simulink model "test1"  (Simulink 10.0)
settings: Solver=VariableStepAuto  StartTime=0.0  StopTime=10.0  RelTol=1e-3
settings Model: Creator=Tan Eng Meng  LastModifiedBy=Tan Eng Meng
settings DataIOCC: SaveFormat=Dataset  ReturnWorkspaceOutputs=on
settings OptimizationCC: LifeSpan=auto
settings DebuggingCC: UnderspecifiedInitializationDetection=Simplified  MergeDetectMultiDrivingBlocksExec=error  SFUnexpectedBacktrackingDiag=error  SFNoUnconditionalDefaultTransitionDiag=error  SFExecutionAtInitializationDiag=warning  ArithmeticOperatorsInVariantConditions=error
settings HardwareCC: ProdBitPerPointer=64  ProdBitPerSizeT=64  ProdBitPerPtrDiffT=64  ProdLargestAtomicFloat=Float  ProdIntDivRoundTo=Zero  ProdEndianess=LittleEndian  ProdWordSize=64  ProdHWDeviceType=Intel->x86-64 (Windows64)
settings ModelReferenceCC: PropagateSignalLabelsOutOfModel=on
settings SFSimCC: SimUseLocalCustomCode=on  CustomCodeUndefinedFunction=FilterOut
settings RTWCC: RTWUseLocalCustomCode=on
settings CodeAppCC: StateflowObjectComments=off
settings GRTTargetCC: TargetLangStandard=C99 (ISO)  CombineOutputUpdateFcns=on  GRTInterface=off
settings ConfigComp: CovMetricSettings=dwe  CovHtmlReporting=off  CovSaveCumulativeToWorkspaceVar=off  CovSaveSingleToWorkspaceVar=off

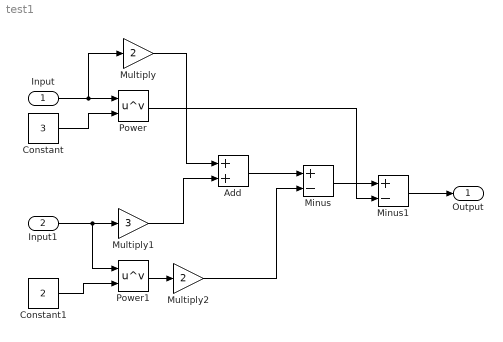
== system test1 ==
  Input : Inport
  Input1 : Inport  Port=2
  Add : Sum
  Constant : Constant  Value=3
  Constant1 : Constant  Value=2
  Minus : Sum  Inputs=+-
  Minus1 : Sum  Inputs=+-
  Multiply : Gain  Gain=2
  Multiply1 : Gain  Gain=3
  Multiply2 : Gain  Gain=2
  Power : Math  Operator=pow  SignedPower=off  SaturateOnIntegerOverflow=on
  Power1 : Math  Operator=pow  SignedPower=off  SaturateOnIntegerOverflow=on
  Output : Outport
  wires:
  Input/1 -> Multiply/1, Power/1
  Constant/1 -> Power/2
  Input1/1 -> Power1/1, Multiply1/1
  Constant1/1 -> Power1/2
  Power1/1 -> Multiply2/1
  Multiply/1 -> Add/1
  Multiply1/1 -> Add/2
  Add/1 -> Minus/1
  Multiply2/1 -> Minus/2
  Minus/1 -> Minus1/1
  Power/1 -> Minus1/2
  Minus1/1 -> Output/1
